simulink model "Suspension_System"  (R2020a)
settings: Solver=VariableStepAuto  StartTime=0.0  StopTime=10.0  RelTol=1e-3
PostLoadFcn:
  | M1=100;
  | M2=10;
  | K1=60;
  | K2=30;
  | b=50;
undefined symbols (not defined in the file): sigbuilder_block
settings Model: DataDictionary=Suspension_data.sldd  Creator=NIKITA  LastModifiedBy=NIKITA

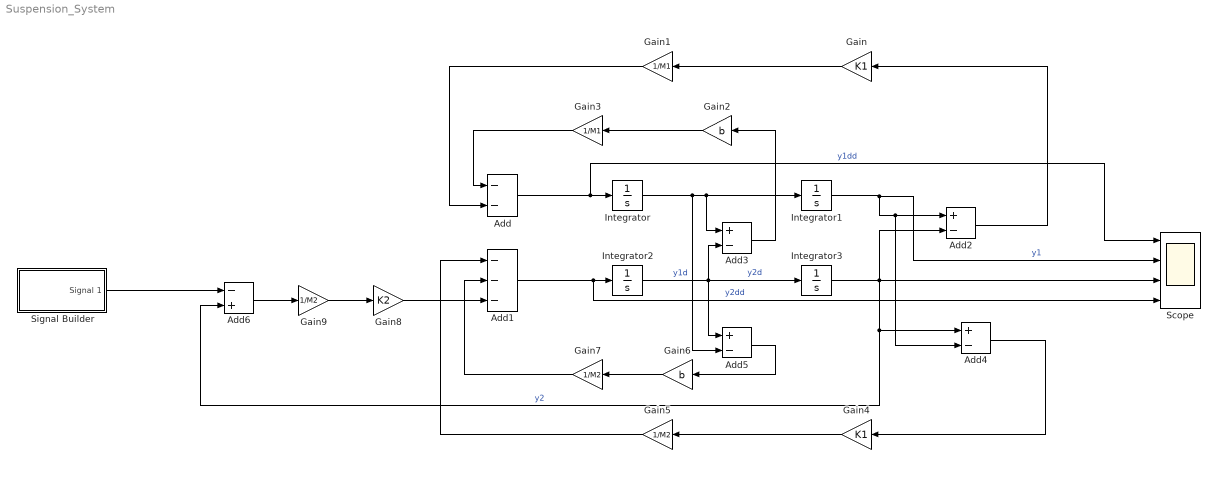
== system Suspension_System ==
  Add : Sum  Inputs=--
  Add1 : Sum  Inputs=---
  Add{2..5} (4 alike) : Sum  Inputs=+-
  Add6 : Sum  Inputs=-+
  Gain : Gain  Gain=K1
  Gain1 : Gain  Gain=1/M1
  Gain2 : Gain  Gain=b
  Gain3 : Gain  Gain=1/M1
  Gain4 : Gain  Gain=K1
  Gain5 : Gain  Gain=1/M2
  Gain6 : Gain  Gain=b
  Gain7 : Gain  Gain=1/M2
  Gain8 : Gain  Gain=K2
  Gain9 : Gain  Gain=1/M2
  Integrator{,1..3} (4 alike) : Integrator
  Scope : Scope  NumInputPorts=4
  Signal Builder : Subsystem  Tag=STV Subsys  LoadFcn=sigbuilder_block('load');  StartFcn=sigbuilder_block('start');  StopFcn=sigbuilder_block('stop');  ClipboardFcn=sigbuilder_block('clipboard');  mask(Sigbuilder block){tuvar=[0:10]}
      mask help: Simulink:masks:SigbuilderBlock_MD
      mask init:
      | if ~strcmp(get_param(bdroot(gcbh),'SimulationStatus'),'stopped') tuvar = sigbuilder_block('maskInit'); end
      settings: CopyFcn=sigbuilder_block('copy');  DeleteFcn=sigbuilder_block('delete');  ModelCloseFcn=sigbuilder_block('modelClose');  PreSaveFcn=sigbuilder_block('preSave');  PauseFcn=sigbuilder_block('pause');  ContinueFcn=sigbuilder_block('continue');  NameChangeFcn=sigbuilder_block('namechange');  OpenFcn=sigbuilder_block('open',[444 157.8 550.8 400.2 ]);  CloseFcn=sigbuilder_block('close');
      mask Display: plot(0, 0, 100, 100,[2, 2, 32, 32, 2], [68, 8, 8, 68, 68],[32, 2], [38, 38], [32, 19, 2],[53, 60, 44], [32, 17, 17, 2],[16, 16, 31, 31]);txt = getActiveGroup(gcbh);text(2, 100, txt,'verticalAlignment', 'top');
  wires:
  Integrator/1 -> Add5/2, Add3/1, Integrator1/1  "y1d"
  Integrator2/1 -> Add5/1, Integrator3/1, Add3/2  "y2d"
  Add/1 -> Scope/1, Integrator/1  "y1dd"
  Add1/1 -> Scope/4, Integrator2/1  "y2dd"
  Integrator1/1 -> Scope/2, Add4/2, Add2/1  "y1"
  Integrator3/1 -> Add2/2, Scope/3, Add6/2, Add4/1  "y2"
  Gain/1 -> Gain1/1
  Add2/1 -> Gain/1
  Add3/1 -> Gain2/1
  Gain2/1 -> Gain3/1
  Gain3/1 -> Add/1
  Gain1/1 -> Add/2
  Add4/1 -> Gain4/1
  Gain4/1 -> Gain5/1
  Gain5/1 -> Add1/1
  Gain6/1 -> Gain7/1
  Add5/1 -> Gain6/1
  Gain7/1 -> Add1/2
  Gain9/1 -> Gain8/1
  Gain8/1 -> Add1/3
  Add6/1 -> Gain9/1
  Signal Builder/1(Signal 1) -> Add6/1

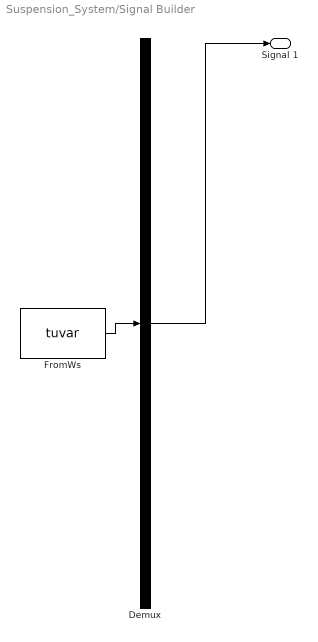
== system Suspension_System/Signal Builder ==
  Demux : Demux  Tag=STV Demux  Outputs=1
      settings: DisplayOption=none
  FromWs : FromWorkspace  Tag=STV FromWs  VariableName=tuvar
      SigBuilderData=|
      | common.afterFinalStr = 'Extrapolate'
      | common.sampleTime = 0
      | dataSet.timeRange = [0 10]
      | dataSet.name = 'Group 1'
      | sbobj.Groups.Name = 'Group 1'
      | sbobj.Groups.Signals.Name = 'Signal 1'
      | sbobj.Groups.Signals.XData = [0 4 4 5.76 5.76 10]
      | sbobj.Groups.Signals.YData = [-0.085 -0.085 0.24 0.63 0.025 0.025]
  Signal 1 : Outport  Tag=STV Outport
  wires:
  Demux/1 -> Signal 1/1
  FromWs/1 -> Demux/1
